simulink model "Final_Dual1"  (R2023a)
settings: Solver=ode113  StartTime=0.0  StopTime=3600  FixedStep=0.01  MaxStep=0.1  RelTol=1e-3
libraries: simulink x3784, slpidlib x2
(part 15 of 158)

== system Final_Dual1/Battery1/Module2/SubModule_4/Cell9 ==
  Cell_Current : Inport
  2RC : Subsystem
  Add : Sum  Inputs=---+
  Lookup Table Dynamic2 : simulink/Lookup Tables/Lookup Table Dynamic  LookUpMeth=Interpolation-Use End Values  OutDataType=fixdt('double')  OutScaling=[]  OutputDataTypeScalingMode=Specify via dialog  OutDataTypeStr=fixdt('double')  DoSatur=off
  Product : Product
  Redution_factor : Constant  Value=[0.8 0.85 0.88 0.95 1 0.98 0.95]
  SOCEstimator : Subsystem  TreatAsAtomicUnit=on
  SOC_Mapping : Subsystem
  Scope : Scope
  Scope1 : Scope
  Scope2 : Scope
  Subsystem : Subsystem
  Temp : Constant  Value=[0 10 20 30 40 50 60]
  Cell_Voltage : Outport
  Cell_temp : Outport  Port=2
  wires:
  2RC/2(V2) -> Add/2
  SOC_Mapping/3(C1) -> 2RC/4(C1)
  SOCEstimator/1(SOC) -> SOC_Mapping/1(SOC), Scope/1
  Add/1 -> Scope2/1, Cell_Voltage/1
  SOC_Mapping/1(Ri) -> Subsystem/2(Ri), 2RC/2(Ri)
  2RC/1(V1) -> Add/1
  2RC/3(Vi) -> Add/3
  Cell_Current/1 -> Subsystem/1(Cell_Current), 2RC/1(Current), SOCEstimator/2(Current)
  SOC_Mapping/2(R1) -> 2RC/3(R1)
  [Cell_Capacity] -> Product/1
  SOC_Mapping/5(C2) -> 2RC/6(C2)
  SOC_Mapping/4(R2) -> 2RC/5(R2)
  [SOC_Iinitial] -> SOCEstimator/1(SOC_Initial)
  SOC_Mapping/6(OCV) -> Add/4
  Subsystem/1(Temp_Cell) -> Scope1/1, SOC_Mapping/2(Cell_Temp), Lookup Table Dynamic2/1, Cell_temp/1
  Product/1 -> SOCEstimator/3(Cell_Capacity)
  Lookup Table Dynamic2/1 -> Product/2
  Temp/1 -> Lookup Table Dynamic2/2
  Redution_factor/1 -> Lookup Table Dynamic2/3

== system Final_Dual1/Battery1/Module2/SubModule_5/Cell1 ==
  Cell_Current : Inport
  2RC : Subsystem
  Add : Sum  Inputs=---+
  Lookup Table Dynamic2 : simulink/Lookup Tables/Lookup Table Dynamic  LookUpMeth=Interpolation-Use End Values  OutDataType=fixdt('double')  OutScaling=[]  OutputDataTypeScalingMode=Specify via dialog  OutDataTypeStr=fixdt('double')  DoSatur=off
  Product : Product
  Redution_factor : Constant  Value=[0.8 0.85 0.88 0.95 1 0.98 0.95]
  SOCEstimator : Subsystem  TreatAsAtomicUnit=on
  SOC_Mapping : Subsystem
  Scope : Scope
  Scope1 : Scope
  Scope2 : Scope
  Subsystem : Subsystem
  Temp : Constant  Value=[0 10 20 30 40 50 60]
  Cell_Voltage : Outport
  Cell_temp : Outport  Port=2
  wires:
  2RC/2(V2) -> Add/2
  SOC_Mapping/3(C1) -> 2RC/4(C1)
  SOCEstimator/1(SOC) -> SOC_Mapping/1(SOC), Scope/1
  Add/1 -> Scope2/1, Cell_Voltage/1
  SOC_Mapping/1(Ri) -> Subsystem/2(Ri), 2RC/2(Ri)
  2RC/1(V1) -> Add/1
  2RC/3(Vi) -> Add/3
  Cell_Current/1 -> Subsystem/1(Cell_Current), 2RC/1(Current), SOCEstimator/2(Current)
  SOC_Mapping/2(R1) -> 2RC/3(R1)
  [Cell_Capacity] -> Product/1
  SOC_Mapping/5(C2) -> 2RC/6(C2)
  SOC_Mapping/4(R2) -> 2RC/5(R2)
  [SOC_Iinitial] -> SOCEstimator/1(SOC_Initial)
  SOC_Mapping/6(OCV) -> Add/4
  Subsystem/1(Temp_Cell) -> Scope1/1, SOC_Mapping/2(Cell_Temp), Lookup Table Dynamic2/1, Cell_temp/1
  Product/1 -> SOCEstimator/3(Cell_Capacity)
  Lookup Table Dynamic2/1 -> Product/2
  Temp/1 -> Lookup Table Dynamic2/2
  Redution_factor/1 -> Lookup Table Dynamic2/3

== system Final_Dual1/Battery1/Module2/SubModule_5/Cell10 ==
  Cell_Current : Inport
  2RC : Subsystem
  Add : Sum  Inputs=---+
  Lookup Table Dynamic2 : simulink/Lookup Tables/Lookup Table Dynamic  LookUpMeth=Interpolation-Use End Values  OutDataType=fixdt('double')  OutScaling=[]  OutputDataTypeScalingMode=Specify via dialog  OutDataTypeStr=fixdt('double')  DoSatur=off
  Product : Product
  Redution_factor : Constant  Value=[0.8 0.85 0.88 0.95 1 0.98 0.95]
  SOCEstimator : Subsystem  TreatAsAtomicUnit=on
  SOC_Mapping : Subsystem
  Scope : Scope
  Scope1 : Scope
  Scope2 : Scope
  Subsystem : Subsystem
  Temp : Constant  Value=[0 10 20 30 40 50 60]
  Cell_Voltage : Outport
  Cell_temp : Outport  Port=2
  wires:
  2RC/2(V2) -> Add/2
  SOC_Mapping/3(C1) -> 2RC/4(C1)
  SOCEstimator/1(SOC) -> SOC_Mapping/1(SOC), Scope/1
  Add/1 -> Scope2/1, Cell_Voltage/1
  SOC_Mapping/1(Ri) -> Subsystem/2(Ri), 2RC/2(Ri)
  2RC/1(V1) -> Add/1
  2RC/3(Vi) -> Add/3
  Cell_Current/1 -> Subsystem/1(Cell_Current), 2RC/1(Current), SOCEstimator/2(Current)
  SOC_Mapping/2(R1) -> 2RC/3(R1)
  [Cell_Capacity] -> Product/1
  SOC_Mapping/5(C2) -> 2RC/6(C2)
  SOC_Mapping/4(R2) -> 2RC/5(R2)
  [SOC_Iinitial] -> SOCEstimator/1(SOC_Initial)
  SOC_Mapping/6(OCV) -> Add/4
  Subsystem/1(Temp_Cell) -> Scope1/1, SOC_Mapping/2(Cell_Temp), Lookup Table Dynamic2/1, Cell_temp/1
  Product/1 -> SOCEstimator/3(Cell_Capacity)
  Lookup Table Dynamic2/1 -> Product/2
  Temp/1 -> Lookup Table Dynamic2/2
  Redution_factor/1 -> Lookup Table Dynamic2/3

== system Final_Dual1/Battery1/Module2/SubModule_5/Cell11 ==
  Cell_Current : Inport
  2RC : Subsystem
  Add : Sum  Inputs=---+
  Lookup Table Dynamic2 : simulink/Lookup Tables/Lookup Table Dynamic  LookUpMeth=Interpolation-Use End Values  OutDataType=fixdt('double')  OutScaling=[]  OutputDataTypeScalingMode=Specify via dialog  OutDataTypeStr=fixdt('double')  DoSatur=off
  Product : Product
  Redution_factor : Constant  Value=[0.8 0.85 0.88 0.95 1 0.98 0.95]
  SOCEstimator : Subsystem  TreatAsAtomicUnit=on
  SOC_Mapping : Subsystem
  Scope : Scope
  Scope1 : Scope
  Scope2 : Scope
  Subsystem : Subsystem
  Temp : Constant  Value=[0 10 20 30 40 50 60]
  Cell_Voltage : Outport
  Cell_temp : Outport  Port=2
  wires:
  Redution_factor/1 -> Lookup Table Dynamic2/3
  Temp/1 -> Lookup Table Dynamic2/2
  Lookup Table Dynamic2/1 -> Product/2
  Product/1 -> SOCEstimator/3(Cell_Capacity)
  Subsystem/1(Temp_Cell) -> Cell_temp/1, Lookup Table Dynamic2/1, SOC_Mapping/2(Cell_Temp), Scope1/1
  SOC_Mapping/6(OCV) -> Add/4
  [SOC_Iinitial] -> SOCEstimator/1(SOC_Initial)
  SOC_Mapping/4(R2) -> 2RC/5(R2)
  SOC_Mapping/5(C2) -> 2RC/6(C2)
  [Cell_Capacity] -> Product/1
  SOC_Mapping/2(R1) -> 2RC/3(R1)
  Cell_Current/1 -> SOCEstimator/2(Current), 2RC/1(Current), Subsystem/1(Cell_Current)
  2RC/3(Vi) -> Add/3
  2RC/1(V1) -> Add/1
  SOC_Mapping/1(Ri) -> 2RC/2(Ri), Subsystem/2(Ri)
  Add/1 -> Cell_Voltage/1, Scope2/1
  SOCEstimator/1(SOC) -> Scope/1, SOC_Mapping/1(SOC)
  SOC_Mapping/3(C1) -> 2RC/4(C1)
  2RC/2(V2) -> Add/2

== system Final_Dual1/Battery1/Module2/SubModule_5/Cell12 ==
  Cell_Current : Inport
  2RC : Subsystem
  Add : Sum  Inputs=---+
  Lookup Table Dynamic2 : simulink/Lookup Tables/Lookup Table Dynamic  LookUpMeth=Interpolation-Use End Values  OutDataType=fixdt('double')  OutScaling=[]  OutputDataTypeScalingMode=Specify via dialog  OutDataTypeStr=fixdt('double')  DoSatur=off
  Product : Product
  Redution_factor : Constant  Value=[0.8 0.85 0.88 0.95 1 0.98 0.95]
  SOCEstimator : Subsystem  TreatAsAtomicUnit=on
  SOC_Mapping : Subsystem
  Scope : Scope
  Scope1 : Scope
  Scope2 : Scope
  Subsystem : Subsystem
  Temp : Constant  Value=[0 10 20 30 40 50 60]
  Cell_Voltage : Outport
  Cell_temp : Outport  Port=2
  wires:
  2RC/2(V2) -> Add/2
  SOC_Mapping/3(C1) -> 2RC/4(C1)
  SOCEstimator/1(SOC) -> SOC_Mapping/1(SOC), Scope/1
  Add/1 -> Scope2/1, Cell_Voltage/1
  SOC_Mapping/1(Ri) -> Subsystem/2(Ri), 2RC/2(Ri)
  2RC/1(V1) -> Add/1
  2RC/3(Vi) -> Add/3
  Cell_Current/1 -> Subsystem/1(Cell_Current), 2RC/1(Current), SOCEstimator/2(Current)
  SOC_Mapping/2(R1) -> 2RC/3(R1)
  [Cell_Capacity] -> Product/1
  SOC_Mapping/5(C2) -> 2RC/6(C2)
  SOC_Mapping/4(R2) -> 2RC/5(R2)
  [SOC_Iinitial] -> SOCEstimator/1(SOC_Initial)
  SOC_Mapping/6(OCV) -> Add/4
  Subsystem/1(Temp_Cell) -> Scope1/1, SOC_Mapping/2(Cell_Temp), Lookup Table Dynamic2/1, Cell_temp/1
  Product/1 -> SOCEstimator/3(Cell_Capacity)
  Lookup Table Dynamic2/1 -> Product/2
  Temp/1 -> Lookup Table Dynamic2/2
  Redution_factor/1 -> Lookup Table Dynamic2/3

== system Final_Dual1/Battery1/Module2/SubModule_5/Cell13 ==
  Cell_Current : Inport
  2RC : Subsystem
  Add : Sum  Inputs=---+
  Lookup Table Dynamic2 : simulink/Lookup Tables/Lookup Table Dynamic  LookUpMeth=Interpolation-Use End Values  OutDataType=fixdt('double')  OutScaling=[]  OutputDataTypeScalingMode=Specify via dialog  OutDataTypeStr=fixdt('double')  DoSatur=off
  Product : Product
  Redution_factor : Constant  Value=[0.8 0.85 0.88 0.95 1 0.98 0.95]
  SOCEstimator : Subsystem  TreatAsAtomicUnit=on
  SOC_Mapping : Subsystem
  Scope : Scope
  Scope1 : Scope
  Scope2 : Scope
  Subsystem : Subsystem
  Temp : Constant  Value=[0 10 20 30 40 50 60]
  Cell_Voltage : Outport
  Cell_temp : Outport  Port=2
  wires:
  Redution_factor/1 -> Lookup Table Dynamic2/3
  Temp/1 -> Lookup Table Dynamic2/2
  Lookup Table Dynamic2/1 -> Product/2
  Product/1 -> SOCEstimator/3(Cell_Capacity)
  Subsystem/1(Temp_Cell) -> Cell_temp/1, Lookup Table Dynamic2/1, SOC_Mapping/2(Cell_Temp), Scope1/1
  SOC_Mapping/6(OCV) -> Add/4
  [SOC_Iinitial] -> SOCEstimator/1(SOC_Initial)
  SOC_Mapping/4(R2) -> 2RC/5(R2)
  SOC_Mapping/5(C2) -> 2RC/6(C2)
  [Cell_Capacity] -> Product/1
  SOC_Mapping/2(R1) -> 2RC/3(R1)
  Cell_Current/1 -> SOCEstimator/2(Current), 2RC/1(Current), Subsystem/1(Cell_Current)
  2RC/3(Vi) -> Add/3
  2RC/1(V1) -> Add/1
  SOC_Mapping/1(Ri) -> 2RC/2(Ri), Subsystem/2(Ri)
  Add/1 -> Cell_Voltage/1, Scope2/1
  SOCEstimator/1(SOC) -> Scope/1, SOC_Mapping/1(SOC)
  SOC_Mapping/3(C1) -> 2RC/4(C1)
  2RC/2(V2) -> Add/2

== system Final_Dual1/Battery1/Module2/SubModule_5/Cell14 ==
  Cell_Current : Inport
  2RC : Subsystem
  Add : Sum  Inputs=---+
  Lookup Table Dynamic2 : simulink/Lookup Tables/Lookup Table Dynamic  LookUpMeth=Interpolation-Use End Values  OutDataType=fixdt('double')  OutScaling=[]  OutputDataTypeScalingMode=Specify via dialog  OutDataTypeStr=fixdt('double')  DoSatur=off
  Product : Product
  Redution_factor : Constant  Value=[0.8 0.85 0.88 0.95 1 0.98 0.95]
  SOCEstimator : Subsystem  TreatAsAtomicUnit=on
  SOC_Mapping : Subsystem
  Scope : Scope
  Scope1 : Scope
  Scope2 : Scope
  Subsystem : Subsystem
  Temp : Constant  Value=[0 10 20 30 40 50 60]
  Cell_Voltage : Outport
  Cell_temp : Outport  Port=2
  wires:
  Redution_factor/1 -> Lookup Table Dynamic2/3
  Temp/1 -> Lookup Table Dynamic2/2
  Lookup Table Dynamic2/1 -> Product/2
  Product/1 -> SOCEstimator/3(Cell_Capacity)
  Subsystem/1(Temp_Cell) -> Cell_temp/1, Lookup Table Dynamic2/1, SOC_Mapping/2(Cell_Temp), Scope1/1
  SOC_Mapping/6(OCV) -> Add/4
  [SOC_Iinitial] -> SOCEstimator/1(SOC_Initial)
  SOC_Mapping/4(R2) -> 2RC/5(R2)
  SOC_Mapping/5(C2) -> 2RC/6(C2)
  [Cell_Capacity] -> Product/1
  SOC_Mapping/2(R1) -> 2RC/3(R1)
  Cell_Current/1 -> SOCEstimator/2(Current), 2RC/1(Current), Subsystem/1(Cell_Current)
  2RC/3(Vi) -> Add/3
  2RC/1(V1) -> Add/1
  SOC_Mapping/1(Ri) -> 2RC/2(Ri), Subsystem/2(Ri)
  Add/1 -> Cell_Voltage/1, Scope2/1
  SOCEstimator/1(SOC) -> Scope/1, SOC_Mapping/1(SOC)
  SOC_Mapping/3(C1) -> 2RC/4(C1)
  2RC/2(V2) -> Add/2

== system Final_Dual1/Battery1/Module2/SubModule_5/Cell15 ==
  Cell_Current : Inport
  2RC : Subsystem
  Add : Sum  Inputs=---+
  Lookup Table Dynamic2 : simulink/Lookup Tables/Lookup Table Dynamic  LookUpMeth=Interpolation-Use End Values  OutDataType=fixdt('double')  OutScaling=[]  OutputDataTypeScalingMode=Specify via dialog  OutDataTypeStr=fixdt('double')  DoSatur=off
  Product : Product
  Redution_factor : Constant  Value=[0.8 0.85 0.88 0.95 1 0.98 0.95]
  SOCEstimator : Subsystem  TreatAsAtomicUnit=on
  SOC_Mapping : Subsystem
  Scope : Scope
  Scope1 : Scope
  Scope2 : Scope
  Subsystem : Subsystem
  Temp : Constant  Value=[0 10 20 30 40 50 60]
  Cell_Voltage : Outport
  Cell_temp : Outport  Port=2
  wires:
  Redution_factor/1 -> Lookup Table Dynamic2/3
  Temp/1 -> Lookup Table Dynamic2/2
  Lookup Table Dynamic2/1 -> Product/2
  Product/1 -> SOCEstimator/3(Cell_Capacity)
  Subsystem/1(Temp_Cell) -> Cell_temp/1, Lookup Table Dynamic2/1, SOC_Mapping/2(Cell_Temp), Scope1/1
  SOC_Mapping/6(OCV) -> Add/4
  [SOC_Iinitial] -> SOCEstimator/1(SOC_Initial)
  SOC_Mapping/4(R2) -> 2RC/5(R2)
  SOC_Mapping/5(C2) -> 2RC/6(C2)
  [Cell_Capacity] -> Product/1
  SOC_Mapping/2(R1) -> 2RC/3(R1)
  Cell_Current/1 -> SOCEstimator/2(Current), 2RC/1(Current), Subsystem/1(Cell_Current)
  2RC/3(Vi) -> Add/3
  2RC/1(V1) -> Add/1
  SOC_Mapping/1(Ri) -> 2RC/2(Ri), Subsystem/2(Ri)
  Add/1 -> Cell_Voltage/1, Scope2/1
  SOCEstimator/1(SOC) -> Scope/1, SOC_Mapping/1(SOC)
  SOC_Mapping/3(C1) -> 2RC/4(C1)
  2RC/2(V2) -> Add/2

== system Final_Dual1/Battery1/Module2/SubModule_5/Cell16 ==
  Cell_Current : Inport
  2RC : Subsystem
  Add : Sum  Inputs=---+
  Lookup Table Dynamic2 : simulink/Lookup Tables/Lookup Table Dynamic  LookUpMeth=Interpolation-Use End Values  OutDataType=fixdt('double')  OutScaling=[]  OutputDataTypeScalingMode=Specify via dialog  OutDataTypeStr=fixdt('double')  DoSatur=off
  Product : Product
  Redution_factor : Constant  Value=[0.8 0.85 0.88 0.95 1 0.98 0.95]
  SOCEstimator : Subsystem  TreatAsAtomicUnit=on
  SOC_Mapping : Subsystem
  Scope : Scope
  Scope1 : Scope
  Scope2 : Scope
  Subsystem : Subsystem
  Temp : Constant  Value=[0 10 20 30 40 50 60]
  Cell_Voltage : Outport
  Cell_temp : Outport  Port=2
  wires:
  Redution_factor/1 -> Lookup Table Dynamic2/3
  Temp/1 -> Lookup Table Dynamic2/2
  Lookup Table Dynamic2/1 -> Product/2
  Product/1 -> SOCEstimator/3(Cell_Capacity)
  Subsystem/1(Temp_Cell) -> Cell_temp/1, Lookup Table Dynamic2/1, SOC_Mapping/2(Cell_Temp), Scope1/1
  SOC_Mapping/6(OCV) -> Add/4
  [SOC_Iinitial] -> SOCEstimator/1(SOC_Initial)
  SOC_Mapping/4(R2) -> 2RC/5(R2)
  SOC_Mapping/5(C2) -> 2RC/6(C2)
  [Cell_Capacity] -> Product/1
  SOC_Mapping/2(R1) -> 2RC/3(R1)
  Cell_Current/1 -> SOCEstimator/2(Current), 2RC/1(Current), Subsystem/1(Cell_Current)
  2RC/3(Vi) -> Add/3
  2RC/1(V1) -> Add/1
  SOC_Mapping/1(Ri) -> 2RC/2(Ri), Subsystem/2(Ri)
  Add/1 -> Cell_Voltage/1, Scope2/1
  SOCEstimator/1(SOC) -> Scope/1, SOC_Mapping/1(SOC)
  SOC_Mapping/3(C1) -> 2RC/4(C1)
  2RC/2(V2) -> Add/2

== system Final_Dual1/Battery1/Module2/SubModule_5/Cell17 ==
  Cell_Current : Inport
  2RC : Subsystem
  Add : Sum  Inputs=---+
  Lookup Table Dynamic2 : simulink/Lookup Tables/Lookup Table Dynamic  LookUpMeth=Interpolation-Use End Values  OutDataType=fixdt('double')  OutScaling=[]  OutputDataTypeScalingMode=Specify via dialog  OutDataTypeStr=fixdt('double')  DoSatur=off
  Product : Product
  Redution_factor : Constant  Value=[0.8 0.85 0.88 0.95 1 0.98 0.95]
  SOCEstimator : Subsystem  TreatAsAtomicUnit=on
  SOC_Mapping : Subsystem
  Scope : Scope
  Scope1 : Scope
  Scope2 : Scope
  Subsystem : Subsystem
  Temp : Constant  Value=[0 10 20 30 40 50 60]
  Cell_Voltage : Outport
  Cell_temp : Outport  Port=2
  wires:
  2RC/2(V2) -> Add/2
  SOC_Mapping/3(C1) -> 2RC/4(C1)
  SOCEstimator/1(SOC) -> SOC_Mapping/1(SOC), Scope/1
  Add/1 -> Scope2/1, Cell_Voltage/1
  SOC_Mapping/1(Ri) -> Subsystem/2(Ri), 2RC/2(Ri)
  2RC/1(V1) -> Add/1
  2RC/3(Vi) -> Add/3
  Cell_Current/1 -> Subsystem/1(Cell_Current), 2RC/1(Current), SOCEstimator/2(Current)
  SOC_Mapping/2(R1) -> 2RC/3(R1)
  [Cell_Capacity] -> Product/1
  SOC_Mapping/5(C2) -> 2RC/6(C2)
  SOC_Mapping/4(R2) -> 2RC/5(R2)
  [SOC_Iinitial] -> SOCEstimator/1(SOC_Initial)
  SOC_Mapping/6(OCV) -> Add/4
  Subsystem/1(Temp_Cell) -> Scope1/1, SOC_Mapping/2(Cell_Temp), Lookup Table Dynamic2/1, Cell_temp/1
  Product/1 -> SOCEstimator/3(Cell_Capacity)
  Lookup Table Dynamic2/1 -> Product/2
  Temp/1 -> Lookup Table Dynamic2/2
  Redution_factor/1 -> Lookup Table Dynamic2/3

== system Final_Dual1/Battery1/Module2/SubModule_5/Cell18 ==
  Cell_Current : Inport
  2RC : Subsystem
  Add : Sum  Inputs=---+
  Lookup Table Dynamic2 : simulink/Lookup Tables/Lookup Table Dynamic  LookUpMeth=Interpolation-Use End Values  OutDataType=fixdt('double')  OutScaling=[]  OutputDataTypeScalingMode=Specify via dialog  OutDataTypeStr=fixdt('double')  DoSatur=off
  Product : Product
  Redution_factor : Constant  Value=[0.8 0.85 0.88 0.95 1 0.98 0.95]
  SOCEstimator : Subsystem  TreatAsAtomicUnit=on
  SOC_Mapping : Subsystem
  Scope : Scope
  Scope1 : Scope
  Scope2 : Scope
  Subsystem : Subsystem
  Temp : Constant  Value=[0 10 20 30 40 50 60]
  Cell_Voltage : Outport
  Cell_temp : Outport  Port=2
  wires:
  Redution_factor/1 -> Lookup Table Dynamic2/3
  Temp/1 -> Lookup Table Dynamic2/2
  Lookup Table Dynamic2/1 -> Product/2
  Product/1 -> SOCEstimator/3(Cell_Capacity)
  Subsystem/1(Temp_Cell) -> Cell_temp/1, Lookup Table Dynamic2/1, SOC_Mapping/2(Cell_Temp), Scope1/1
  SOC_Mapping/6(OCV) -> Add/4
  [SOC_Iinitial] -> SOCEstimator/1(SOC_Initial)
  SOC_Mapping/4(R2) -> 2RC/5(R2)
  SOC_Mapping/5(C2) -> 2RC/6(C2)
  [Cell_Capacity] -> Product/1
  SOC_Mapping/2(R1) -> 2RC/3(R1)
  Cell_Current/1 -> SOCEstimator/2(Current), 2RC/1(Current), Subsystem/1(Cell_Current)
  2RC/3(Vi) -> Add/3
  2RC/1(V1) -> Add/1
  SOC_Mapping/1(Ri) -> 2RC/2(Ri), Subsystem/2(Ri)
  Add/1 -> Cell_Voltage/1, Scope2/1
  SOCEstimator/1(SOC) -> Scope/1, SOC_Mapping/1(SOC)
  SOC_Mapping/3(C1) -> 2RC/4(C1)
  2RC/2(V2) -> Add/2

== system Final_Dual1/Battery1/Module2/SubModule_5/Cell19 ==
  Cell_Current : Inport
  2RC : Subsystem
  Add : Sum  Inputs=---+
  Lookup Table Dynamic2 : simulink/Lookup Tables/Lookup Table Dynamic  LookUpMeth=Interpolation-Use End Values  OutDataType=fixdt('double')  OutScaling=[]  OutputDataTypeScalingMode=Specify via dialog  OutDataTypeStr=fixdt('double')  DoSatur=off
  Product : Product
  Redution_factor : Constant  Value=[0.8 0.85 0.88 0.95 1 0.98 0.95]
  SOCEstimator : Subsystem  TreatAsAtomicUnit=on
  SOC_Mapping : Subsystem
  Scope : Scope
  Scope1 : Scope
  Scope2 : Scope
  Subsystem : Subsystem
  Temp : Constant  Value=[0 10 20 30 40 50 60]
  Cell_Voltage : Outport
  Cell_temp : Outport  Port=2
  wires:
  2RC/2(V2) -> Add/2
  SOC_Mapping/3(C1) -> 2RC/4(C1)
  SOCEstimator/1(SOC) -> SOC_Mapping/1(SOC), Scope/1
  Add/1 -> Scope2/1, Cell_Voltage/1
  SOC_Mapping/1(Ri) -> Subsystem/2(Ri), 2RC/2(Ri)
  2RC/1(V1) -> Add/1
  2RC/3(Vi) -> Add/3
  Cell_Current/1 -> Subsystem/1(Cell_Current), 2RC/1(Current), SOCEstimator/2(Current)
  SOC_Mapping/2(R1) -> 2RC/3(R1)
  [Cell_Capacity] -> Product/1
  SOC_Mapping/5(C2) -> 2RC/6(C2)
  SOC_Mapping/4(R2) -> 2RC/5(R2)
  [SOC_Iinitial] -> SOCEstimator/1(SOC_Initial)
  SOC_Mapping/6(OCV) -> Add/4
  Subsystem/1(Temp_Cell) -> Scope1/1, SOC_Mapping/2(Cell_Temp), Lookup Table Dynamic2/1, Cell_temp/1
  Product/1 -> SOCEstimator/3(Cell_Capacity)
  Lookup Table Dynamic2/1 -> Product/2
  Temp/1 -> Lookup Table Dynamic2/2
  Redution_factor/1 -> Lookup Table Dynamic2/3

== system Final_Dual1/Battery1/Module2/SubModule_5/Cell2 ==
  Cell_Current : Inport
  2RC : Subsystem
  Add : Sum  Inputs=---+
  Lookup Table Dynamic2 : simulink/Lookup Tables/Lookup Table Dynamic  LookUpMeth=Interpolation-Use End Values  OutDataType=fixdt('double')  OutScaling=[]  OutputDataTypeScalingMode=Specify via dialog  OutDataTypeStr=fixdt('double')  DoSatur=off
  Product : Product
  Redution_factor : Constant  Value=[0.8 0.85 0.88 0.95 1 0.98 0.95]
  SOCEstimator : Subsystem  TreatAsAtomicUnit=on
  SOC_Mapping : Subsystem
  Scope : Scope
  Scope1 : Scope
  Scope2 : Scope
  Subsystem : Subsystem
  Temp : Constant  Value=[0 10 20 30 40 50 60]
  Cell_Voltage : Outport
  Cell_temp : Outport  Port=2
  wires:
  Redution_factor/1 -> Lookup Table Dynamic2/3
  Temp/1 -> Lookup Table Dynamic2/2
  Lookup Table Dynamic2/1 -> Product/2
  Product/1 -> SOCEstimator/3(Cell_Capacity)
  Subsystem/1(Temp_Cell) -> Cell_temp/1, Lookup Table Dynamic2/1, SOC_Mapping/2(Cell_Temp), Scope1/1
  SOC_Mapping/6(OCV) -> Add/4
  [SOC_Iinitial] -> SOCEstimator/1(SOC_Initial)
  SOC_Mapping/4(R2) -> 2RC/5(R2)
  SOC_Mapping/5(C2) -> 2RC/6(C2)
  [Cell_Capacity] -> Product/1
  SOC_Mapping/2(R1) -> 2RC/3(R1)
  Cell_Current/1 -> SOCEstimator/2(Current), 2RC/1(Current), Subsystem/1(Cell_Current)
  2RC/3(Vi) -> Add/3
  2RC/1(V1) -> Add/1
  SOC_Mapping/1(Ri) -> 2RC/2(Ri), Subsystem/2(Ri)
  Add/1 -> Cell_Voltage/1, Scope2/1
  SOCEstimator/1(SOC) -> Scope/1, SOC_Mapping/1(SOC)
  SOC_Mapping/3(C1) -> 2RC/4(C1)
  2RC/2(V2) -> Add/2

== system Final_Dual1/Battery1/Module2/SubModule_5/Cell20 ==
  Cell_Current : Inport
  2RC : Subsystem
  Add : Sum  Inputs=---+
  Lookup Table Dynamic2 : simulink/Lookup Tables/Lookup Table Dynamic  LookUpMeth=Interpolation-Use End Values  OutDataType=fixdt('double')  OutScaling=[]  OutputDataTypeScalingMode=Specify via dialog  OutDataTypeStr=fixdt('double')  DoSatur=off
  Product : Product
  Redution_factor : Constant  Value=[0.8 0.85 0.88 0.95 1 0.98 0.95]
  SOCEstimator : Subsystem  TreatAsAtomicUnit=on
  SOC_Mapping : Subsystem
  Scope : Scope
  Scope1 : Scope
  Scope2 : Scope
  Subsystem : Subsystem
  Temp : Constant  Value=[0 10 20 30 40 50 60]
  Cell_Voltage : Outport
  Cell_temp : Outport  Port=2
  wires:
  Redution_factor/1 -> Lookup Table Dynamic2/3
  Temp/1 -> Lookup Table Dynamic2/2
  Lookup Table Dynamic2/1 -> Product/2
  Product/1 -> SOCEstimator/3(Cell_Capacity)
  Subsystem/1(Temp_Cell) -> Cell_temp/1, Lookup Table Dynamic2/1, SOC_Mapping/2(Cell_Temp), Scope1/1
  SOC_Mapping/6(OCV) -> Add/4
  [SOC_Iinitial] -> SOCEstimator/1(SOC_Initial)
  SOC_Mapping/4(R2) -> 2RC/5(R2)
  SOC_Mapping/5(C2) -> 2RC/6(C2)
  [Cell_Capacity] -> Product/1
  SOC_Mapping/2(R1) -> 2RC/3(R1)
  Cell_Current/1 -> SOCEstimator/2(Current), 2RC/1(Current), Subsystem/1(Cell_Current)
  2RC/3(Vi) -> Add/3
  2RC/1(V1) -> Add/1
  SOC_Mapping/1(Ri) -> 2RC/2(Ri), Subsystem/2(Ri)
  Add/1 -> Cell_Voltage/1, Scope2/1
  SOCEstimator/1(SOC) -> Scope/1, SOC_Mapping/1(SOC)
  SOC_Mapping/3(C1) -> 2RC/4(C1)
  2RC/2(V2) -> Add/2

== system Final_Dual1/Battery1/Module2/SubModule_5/Cell21 ==
  Cell_Current : Inport
  2RC : Subsystem
  Add : Sum  Inputs=---+
  Lookup Table Dynamic2 : simulink/Lookup Tables/Lookup Table Dynamic  LookUpMeth=Interpolation-Use End Values  OutDataType=fixdt('double')  OutScaling=[]  OutputDataTypeScalingMode=Specify via dialog  OutDataTypeStr=fixdt('double')  DoSatur=off
  Product : Product
  Redution_factor : Constant  Value=[0.8 0.85 0.88 0.95 1 0.98 0.95]
  SOCEstimator : Subsystem  TreatAsAtomicUnit=on
  SOC_Mapping : Subsystem
  Scope : Scope
  Scope1 : Scope
  Scope2 : Scope
  Subsystem : Subsystem
  Temp : Constant  Value=[0 10 20 30 40 50 60]
  Cell_Voltage : Outport
  Cell_temp : Outport  Port=2
  wires:
  2RC/2(V2) -> Add/2
  SOC_Mapping/3(C1) -> 2RC/4(C1)
  SOCEstimator/1(SOC) -> SOC_Mapping/1(SOC), Scope/1
  Add/1 -> Scope2/1, Cell_Voltage/1
  SOC_Mapping/1(Ri) -> Subsystem/2(Ri), 2RC/2(Ri)
  2RC/1(V1) -> Add/1
  2RC/3(Vi) -> Add/3
  Cell_Current/1 -> Subsystem/1(Cell_Current), 2RC/1(Current), SOCEstimator/2(Current)
  SOC_Mapping/2(R1) -> 2RC/3(R1)
  [Cell_Capacity] -> Product/1
  SOC_Mapping/5(C2) -> 2RC/6(C2)
  SOC_Mapping/4(R2) -> 2RC/5(R2)
  [SOC_Iinitial] -> SOCEstimator/1(SOC_Initial)
  SOC_Mapping/6(OCV) -> Add/4
  Subsystem/1(Temp_Cell) -> Scope1/1, SOC_Mapping/2(Cell_Temp), Lookup Table Dynamic2/1, Cell_temp/1
  Product/1 -> SOCEstimator/3(Cell_Capacity)
  Lookup Table Dynamic2/1 -> Product/2
  Temp/1 -> Lookup Table Dynamic2/2
  Redution_factor/1 -> Lookup Table Dynamic2/3

== system Final_Dual1/Battery1/Module2/SubModule_5/Cell22 ==
  Cell_Current : Inport
  2RC : Subsystem
  Add : Sum  Inputs=---+
  Lookup Table Dynamic2 : simulink/Lookup Tables/Lookup Table Dynamic  LookUpMeth=Interpolation-Use End Values  OutDataType=fixdt('double')  OutScaling=[]  OutputDataTypeScalingMode=Specify via dialog  OutDataTypeStr=fixdt('double')  DoSatur=off
  Product : Product
  Redution_factor : Constant  Value=[0.8 0.85 0.88 0.95 1 0.98 0.95]
  SOCEstimator : Subsystem  TreatAsAtomicUnit=on
  SOC_Mapping : Subsystem
  Scope : Scope
  Scope1 : Scope
  Scope2 : Scope
  Subsystem : Subsystem
  Temp : Constant  Value=[0 10 20 30 40 50 60]
  Cell_Voltage : Outport
  Cell_temp : Outport  Port=2
  wires:
  2RC/2(V2) -> Add/2
  SOC_Mapping/3(C1) -> 2RC/4(C1)
  SOCEstimator/1(SOC) -> SOC_Mapping/1(SOC), Scope/1
  Add/1 -> Scope2/1, Cell_Voltage/1
  SOC_Mapping/1(Ri) -> Subsystem/2(Ri), 2RC/2(Ri)
  2RC/1(V1) -> Add/1
  2RC/3(Vi) -> Add/3
  Cell_Current/1 -> Subsystem/1(Cell_Current), 2RC/1(Current), SOCEstimator/2(Current)
  SOC_Mapping/2(R1) -> 2RC/3(R1)
  [Cell_Capacity] -> Product/1
  SOC_Mapping/5(C2) -> 2RC/6(C2)
  SOC_Mapping/4(R2) -> 2RC/5(R2)
  [SOC_Iinitial] -> SOCEstimator/1(SOC_Initial)
  SOC_Mapping/6(OCV) -> Add/4
  Subsystem/1(Temp_Cell) -> Scope1/1, SOC_Mapping/2(Cell_Temp), Lookup Table Dynamic2/1, Cell_temp/1
  Product/1 -> SOCEstimator/3(Cell_Capacity)
  Lookup Table Dynamic2/1 -> Product/2
  Temp/1 -> Lookup Table Dynamic2/2
  Redution_factor/1 -> Lookup Table Dynamic2/3

== system Final_Dual1/Battery1/Module2/SubModule_5/Cell3 ==
  Cell_Current : Inport
  2RC : Subsystem
  Add : Sum  Inputs=---+
  Lookup Table Dynamic2 : simulink/Lookup Tables/Lookup Table Dynamic  LookUpMeth=Interpolation-Use End Values  OutDataType=fixdt('double')  OutScaling=[]  OutputDataTypeScalingMode=Specify via dialog  OutDataTypeStr=fixdt('double')  DoSatur=off
  Product : Product
  Redution_factor : Constant  Value=[0.8 0.85 0.88 0.95 1 0.98 0.95]
  SOCEstimator : Subsystem  TreatAsAtomicUnit=on
  SOC_Mapping : Subsystem
  Scope : Scope
  Scope1 : Scope
  Scope2 : Scope
  Subsystem : Subsystem
  Temp : Constant  Value=[0 10 20 30 40 50 60]
  Cell_Voltage : Outport
  Cell_temp : Outport  Port=2
  wires:
  2RC/2(V2) -> Add/2
  SOC_Mapping/3(C1) -> 2RC/4(C1)
  SOCEstimator/1(SOC) -> SOC_Mapping/1(SOC), Scope/1
  Add/1 -> Scope2/1, Cell_Voltage/1
  SOC_Mapping/1(Ri) -> Subsystem/2(Ri), 2RC/2(Ri)
  2RC/1(V1) -> Add/1
  2RC/3(Vi) -> Add/3
  Cell_Current/1 -> Subsystem/1(Cell_Current), 2RC/1(Current), SOCEstimator/2(Current)
  SOC_Mapping/2(R1) -> 2RC/3(R1)
  [Cell_Capacity] -> Product/1
  SOC_Mapping/5(C2) -> 2RC/6(C2)
  SOC_Mapping/4(R2) -> 2RC/5(R2)
  [SOC_Iinitial] -> SOCEstimator/1(SOC_Initial)
  SOC_Mapping/6(OCV) -> Add/4
  Subsystem/1(Temp_Cell) -> Scope1/1, SOC_Mapping/2(Cell_Temp), Lookup Table Dynamic2/1, Cell_temp/1
  Product/1 -> SOCEstimator/3(Cell_Capacity)
  Lookup Table Dynamic2/1 -> Product/2
  Temp/1 -> Lookup Table Dynamic2/2
  Redution_factor/1 -> Lookup Table Dynamic2/3

== system Final_Dual1/Battery1/Module2/SubModule_5/Cell4 ==
  Cell_Current : Inport
  2RC : Subsystem
  Add : Sum  Inputs=---+
  Lookup Table Dynamic2 : simulink/Lookup Tables/Lookup Table Dynamic  LookUpMeth=Interpolation-Use End Values  OutDataType=fixdt('double')  OutScaling=[]  OutputDataTypeScalingMode=Specify via dialog  OutDataTypeStr=fixdt('double')  DoSatur=off
  Product : Product
  Redution_factor : Constant  Value=[0.8 0.85 0.88 0.95 1 0.98 0.95]
  SOCEstimator : Subsystem  TreatAsAtomicUnit=on
  SOC_Mapping : Subsystem
  Scope : Scope
  Scope1 : Scope
  Scope2 : Scope
  Subsystem : Subsystem
  Temp : Constant  Value=[0 10 20 30 40 50 60]
  Cell_Voltage : Outport
  Cell_temp : Outport  Port=2
  wires:
  Redution_factor/1 -> Lookup Table Dynamic2/3
  Temp/1 -> Lookup Table Dynamic2/2
  Lookup Table Dynamic2/1 -> Product/2
  Product/1 -> SOCEstimator/3(Cell_Capacity)
  Subsystem/1(Temp_Cell) -> Cell_temp/1, Lookup Table Dynamic2/1, SOC_Mapping/2(Cell_Temp), Scope1/1
  SOC_Mapping/6(OCV) -> Add/4
  [SOC_Iinitial] -> SOCEstimator/1(SOC_Initial)
  SOC_Mapping/4(R2) -> 2RC/5(R2)
  SOC_Mapping/5(C2) -> 2RC/6(C2)
  [Cell_Capacity] -> Product/1
  SOC_Mapping/2(R1) -> 2RC/3(R1)
  Cell_Current/1 -> SOCEstimator/2(Current), 2RC/1(Current), Subsystem/1(Cell_Current)
  2RC/3(Vi) -> Add/3
  2RC/1(V1) -> Add/1
  SOC_Mapping/1(Ri) -> 2RC/2(Ri), Subsystem/2(Ri)
  Add/1 -> Cell_Voltage/1, Scope2/1
  SOCEstimator/1(SOC) -> Scope/1, SOC_Mapping/1(SOC)
  SOC_Mapping/3(C1) -> 2RC/4(C1)
  2RC/2(V2) -> Add/2

== system Final_Dual1/Battery1/Module2/SubModule_5/Cell5 ==
  Cell_Current : Inport
  2RC : Subsystem
  Add : Sum  Inputs=---+
  Lookup Table Dynamic2 : simulink/Lookup Tables/Lookup Table Dynamic  LookUpMeth=Interpolation-Use End Values  OutDataType=fixdt('double')  OutScaling=[]  OutputDataTypeScalingMode=Specify via dialog  OutDataTypeStr=fixdt('double')  DoSatur=off
  Product : Product
  Redution_factor : Constant  Value=[0.8 0.85 0.88 0.95 1 0.98 0.95]
  SOCEstimator : Subsystem  TreatAsAtomicUnit=on
  SOC_Mapping : Subsystem
  Scope : Scope
  Scope1 : Scope
  Scope2 : Scope
  Subsystem : Subsystem
  Temp : Constant  Value=[0 10 20 30 40 50 60]
  Cell_Voltage : Outport
  Cell_temp : Outport  Port=2
  wires:
  2RC/2(V2) -> Add/2
  SOC_Mapping/3(C1) -> 2RC/4(C1)
  SOCEstimator/1(SOC) -> SOC_Mapping/1(SOC), Scope/1
  Add/1 -> Scope2/1, Cell_Voltage/1
  SOC_Mapping/1(Ri) -> Subsystem/2(Ri), 2RC/2(Ri)
  2RC/1(V1) -> Add/1
  2RC/3(Vi) -> Add/3
  Cell_Current/1 -> Subsystem/1(Cell_Current), 2RC/1(Current), SOCEstimator/2(Current)
  SOC_Mapping/2(R1) -> 2RC/3(R1)
  [Cell_Capacity] -> Product/1
  SOC_Mapping/5(C2) -> 2RC/6(C2)
  SOC_Mapping/4(R2) -> 2RC/5(R2)
  [SOC_Iinitial] -> SOCEstimator/1(SOC_Initial)
  SOC_Mapping/6(OCV) -> Add/4
  Subsystem/1(Temp_Cell) -> Scope1/1, SOC_Mapping/2(Cell_Temp), Lookup Table Dynamic2/1, Cell_temp/1
  Product/1 -> SOCEstimator/3(Cell_Capacity)
  Lookup Table Dynamic2/1 -> Product/2
  Temp/1 -> Lookup Table Dynamic2/2
  Redution_factor/1 -> Lookup Table Dynamic2/3

== system Final_Dual1/Battery1/Module2/SubModule_5/Cell6 ==
  Cell_Current : Inport
  2RC : Subsystem
  Add : Sum  Inputs=---+
  Lookup Table Dynamic2 : simulink/Lookup Tables/Lookup Table Dynamic  LookUpMeth=Interpolation-Use End Values  OutDataType=fixdt('double')  OutScaling=[]  OutputDataTypeScalingMode=Specify via dialog  OutDataTypeStr=fixdt('double')  DoSatur=off
  Product : Product
  Redution_factor : Constant  Value=[0.8 0.85 0.88 0.95 1 0.98 0.95]
  SOCEstimator : Subsystem  TreatAsAtomicUnit=on
  SOC_Mapping : Subsystem
  Scope : Scope
  Scope1 : Scope
  Scope2 : Scope
  Subsystem : Subsystem
  Temp : Constant  Value=[0 10 20 30 40 50 60]
  Cell_Voltage : Outport
  Cell_temp : Outport  Port=2
  wires:
  Redution_factor/1 -> Lookup Table Dynamic2/3
  Temp/1 -> Lookup Table Dynamic2/2
  Lookup Table Dynamic2/1 -> Product/2
  Product/1 -> SOCEstimator/3(Cell_Capacity)
  Subsystem/1(Temp_Cell) -> Cell_temp/1, Lookup Table Dynamic2/1, SOC_Mapping/2(Cell_Temp), Scope1/1
  SOC_Mapping/6(OCV) -> Add/4
  [SOC_Iinitial] -> SOCEstimator/1(SOC_Initial)
  SOC_Mapping/4(R2) -> 2RC/5(R2)
  SOC_Mapping/5(C2) -> 2RC/6(C2)
  [Cell_Capacity] -> Product/1
  SOC_Mapping/2(R1) -> 2RC/3(R1)
  Cell_Current/1 -> SOCEstimator/2(Current), 2RC/1(Current), Subsystem/1(Cell_Current)
  2RC/3(Vi) -> Add/3
  2RC/1(V1) -> Add/1
  SOC_Mapping/1(Ri) -> 2RC/2(Ri), Subsystem/2(Ri)
  Add/1 -> Cell_Voltage/1, Scope2/1
  SOCEstimator/1(SOC) -> Scope/1, SOC_Mapping/1(SOC)
  SOC_Mapping/3(C1) -> 2RC/4(C1)
  2RC/2(V2) -> Add/2

== system Final_Dual1/Battery1/Module2/SubModule_5/Cell7 ==
  Cell_Current : Inport
  2RC : Subsystem
  Add : Sum  Inputs=---+
  Lookup Table Dynamic2 : simulink/Lookup Tables/Lookup Table Dynamic  LookUpMeth=Interpolation-Use End Values  OutDataType=fixdt('double')  OutScaling=[]  OutputDataTypeScalingMode=Specify via dialog  OutDataTypeStr=fixdt('double')  DoSatur=off
  Product : Product
  Redution_factor : Constant  Value=[0.8 0.85 0.88 0.95 1 0.98 0.95]
  SOCEstimator : Subsystem  TreatAsAtomicUnit=on
  SOC_Mapping : Subsystem
  Scope : Scope
  Scope1 : Scope
  Scope2 : Scope
  Subsystem : Subsystem
  Temp : Constant  Value=[0 10 20 30 40 50 60]
  Cell_Voltage : Outport
  Cell_temp : Outport  Port=2
  wires:
  Redution_factor/1 -> Lookup Table Dynamic2/3
  Temp/1 -> Lookup Table Dynamic2/2
  Lookup Table Dynamic2/1 -> Product/2
  Product/1 -> SOCEstimator/3(Cell_Capacity)
  Subsystem/1(Temp_Cell) -> Cell_temp/1, Lookup Table Dynamic2/1, SOC_Mapping/2(Cell_Temp), Scope1/1
  SOC_Mapping/6(OCV) -> Add/4
  [SOC_Iinitial] -> SOCEstimator/1(SOC_Initial)
  SOC_Mapping/4(R2) -> 2RC/5(R2)
  SOC_Mapping/5(C2) -> 2RC/6(C2)
  [Cell_Capacity] -> Product/1
  SOC_Mapping/2(R1) -> 2RC/3(R1)
  Cell_Current/1 -> SOCEstimator/2(Current), 2RC/1(Current), Subsystem/1(Cell_Current)
  2RC/3(Vi) -> Add/3
  2RC/1(V1) -> Add/1
  SOC_Mapping/1(Ri) -> 2RC/2(Ri), Subsystem/2(Ri)
  Add/1 -> Cell_Voltage/1, Scope2/1
  SOCEstimator/1(SOC) -> Scope/1, SOC_Mapping/1(SOC)
  SOC_Mapping/3(C1) -> 2RC/4(C1)
  2RC/2(V2) -> Add/2

== system Final_Dual1/Battery1/Module2/SubModule_5/Cell8 ==
  Cell_Current : Inport
  2RC : Subsystem
  Add : Sum  Inputs=---+
  Lookup Table Dynamic2 : simulink/Lookup Tables/Lookup Table Dynamic  LookUpMeth=Interpolation-Use End Values  OutDataType=fixdt('double')  OutScaling=[]  OutputDataTypeScalingMode=Specify via dialog  OutDataTypeStr=fixdt('double')  DoSatur=off
  Product : Product
  Redution_factor : Constant  Value=[0.8 0.85 0.88 0.95 1 0.98 0.95]
  SOCEstimator : Subsystem  TreatAsAtomicUnit=on
  SOC_Mapping : Subsystem
  Scope : Scope
  Scope1 : Scope
  Scope2 : Scope
  Subsystem : Subsystem
  Temp : Constant  Value=[0 10 20 30 40 50 60]
  Cell_Voltage : Outport
  Cell_temp : Outport  Port=2
  wires:
  2RC/2(V2) -> Add/2
  SOC_Mapping/3(C1) -> 2RC/4(C1)
  SOCEstimator/1(SOC) -> SOC_Mapping/1(SOC), Scope/1
  Add/1 -> Scope2/1, Cell_Voltage/1
  SOC_Mapping/1(Ri) -> Subsystem/2(Ri), 2RC/2(Ri)
  2RC/1(V1) -> Add/1
  2RC/3(Vi) -> Add/3
  Cell_Current/1 -> Subsystem/1(Cell_Current), 2RC/1(Current), SOCEstimator/2(Current)
  SOC_Mapping/2(R1) -> 2RC/3(R1)
  [Cell_Capacity] -> Product/1
  SOC_Mapping/5(C2) -> 2RC/6(C2)
  SOC_Mapping/4(R2) -> 2RC/5(R2)
  [SOC_Iinitial] -> SOCEstimator/1(SOC_Initial)
  SOC_Mapping/6(OCV) -> Add/4
  Subsystem/1(Temp_Cell) -> Scope1/1, SOC_Mapping/2(Cell_Temp), Lookup Table Dynamic2/1, Cell_temp/1
  Product/1 -> SOCEstimator/3(Cell_Capacity)
  Lookup Table Dynamic2/1 -> Product/2
  Temp/1 -> Lookup Table Dynamic2/2
  Redution_factor/1 -> Lookup Table Dynamic2/3

== system Final_Dual1/Battery1/Module2/SubModule_5/Cell9 ==
  Cell_Current : Inport
  2RC : Subsystem
  Add : Sum  Inputs=---+
  Lookup Table Dynamic2 : simulink/Lookup Tables/Lookup Table Dynamic  LookUpMeth=Interpolation-Use End Values  OutDataType=fixdt('double')  OutScaling=[]  OutputDataTypeScalingMode=Specify via dialog  OutDataTypeStr=fixdt('double')  DoSatur=off
  Product : Product
  Redution_factor : Constant  Value=[0.8 0.85 0.88 0.95 1 0.98 0.95]
  SOCEstimator : Subsystem  TreatAsAtomicUnit=on
  SOC_Mapping : Subsystem
  Scope : Scope
  Scope1 : Scope
  Scope2 : Scope
  Subsystem : Subsystem
  Temp : Constant  Value=[0 10 20 30 40 50 60]
  Cell_Voltage : Outport
  Cell_temp : Outport  Port=2
  wires:
  Redution_factor/1 -> Lookup Table Dynamic2/3
  Temp/1 -> Lookup Table Dynamic2/2
  Lookup Table Dynamic2/1 -> Product/2
  Product/1 -> SOCEstimator/3(Cell_Capacity)
  Subsystem/1(Temp_Cell) -> Cell_temp/1, Lookup Table Dynamic2/1, SOC_Mapping/2(Cell_Temp), Scope1/1
  SOC_Mapping/6(OCV) -> Add/4
  [SOC_Iinitial] -> SOCEstimator/1(SOC_Initial)
  SOC_Mapping/4(R2) -> 2RC/5(R2)
  SOC_Mapping/5(C2) -> 2RC/6(C2)
  [Cell_Capacity] -> Product/1
  SOC_Mapping/2(R1) -> 2RC/3(R1)
  Cell_Current/1 -> SOCEstimator/2(Current), 2RC/1(Current), Subsystem/1(Cell_Current)
  2RC/3(Vi) -> Add/3
  2RC/1(V1) -> Add/1
  SOC_Mapping/1(Ri) -> 2RC/2(Ri), Subsystem/2(Ri)
  Add/1 -> Cell_Voltage/1, Scope2/1
  SOCEstimator/1(SOC) -> Scope/1, SOC_Mapping/1(SOC)
  SOC_Mapping/3(C1) -> 2RC/4(C1)
  2RC/2(V2) -> Add/2

== system Final_Dual1/Battery1/Module2/SubModule_6/Cell1 ==
  Cell_Current : Inport
  2RC : Subsystem
  Add : Sum  Inputs=---+
  Lookup Table Dynamic2 : simulink/Lookup Tables/Lookup Table Dynamic  LookUpMeth=Interpolation-Use End Values  OutDataType=fixdt('double')  OutScaling=[]  OutputDataTypeScalingMode=Specify via dialog  OutDataTypeStr=fixdt('double')  DoSatur=off
  Product : Product
  Redution_factor : Constant  Value=[0.8 0.85 0.88 0.95 1 0.98 0.95]
  SOCEstimator : Subsystem  TreatAsAtomicUnit=on
  SOC_Mapping : Subsystem
  Scope : Scope
  Scope1 : Scope
  Scope2 : Scope
  Subsystem : Subsystem
  Temp : Constant  Value=[0 10 20 30 40 50 60]
  Cell_Voltage : Outport
  Cell_temp : Outport  Port=2
  wires:
  Redution_factor/1 -> Lookup Table Dynamic2/3
  Temp/1 -> Lookup Table Dynamic2/2
  Lookup Table Dynamic2/1 -> Product/2
  Product/1 -> SOCEstimator/3(Cell_Capacity)
  Subsystem/1(Temp_Cell) -> Cell_temp/1, Lookup Table Dynamic2/1, SOC_Mapping/2(Cell_Temp), Scope1/1
  SOC_Mapping/6(OCV) -> Add/4
  [SOC_Iinitial] -> SOCEstimator/1(SOC_Initial)
  SOC_Mapping/4(R2) -> 2RC/5(R2)
  SOC_Mapping/5(C2) -> 2RC/6(C2)
  [Cell_Capacity] -> Product/1
  SOC_Mapping/2(R1) -> 2RC/3(R1)
  Cell_Current/1 -> SOCEstimator/2(Current), 2RC/1(Current), Subsystem/1(Cell_Current)
  2RC/3(Vi) -> Add/3
  2RC/1(V1) -> Add/1
  SOC_Mapping/1(Ri) -> 2RC/2(Ri), Subsystem/2(Ri)
  Add/1 -> Cell_Voltage/1, Scope2/1
  SOCEstimator/1(SOC) -> Scope/1, SOC_Mapping/1(SOC)
  SOC_Mapping/3(C1) -> 2RC/4(C1)
  2RC/2(V2) -> Add/2

== system Final_Dual1/Battery1/Module2/SubModule_6/Cell10 ==
  Cell_Current : Inport
  2RC : Subsystem
  Add : Sum  Inputs=---+
  Lookup Table Dynamic2 : simulink/Lookup Tables/Lookup Table Dynamic  LookUpMeth=Interpolation-Use End Values  OutDataType=fixdt('double')  OutScaling=[]  OutputDataTypeScalingMode=Specify via dialog  OutDataTypeStr=fixdt('double')  DoSatur=off
  Product : Product
  Redution_factor : Constant  Value=[0.8 0.85 0.88 0.95 1 0.98 0.95]
  SOCEstimator : Subsystem  TreatAsAtomicUnit=on
  SOC_Mapping : Subsystem
  Scope : Scope
  Scope1 : Scope
  Scope2 : Scope
  Subsystem : Subsystem
  Temp : Constant  Value=[0 10 20 30 40 50 60]
  Cell_Voltage : Outport
  Cell_temp : Outport  Port=2
  wires:
  Redution_factor/1 -> Lookup Table Dynamic2/3
  Temp/1 -> Lookup Table Dynamic2/2
  Lookup Table Dynamic2/1 -> Product/2
  Product/1 -> SOCEstimator/3(Cell_Capacity)
  Subsystem/1(Temp_Cell) -> Cell_temp/1, Lookup Table Dynamic2/1, SOC_Mapping/2(Cell_Temp), Scope1/1
  SOC_Mapping/6(OCV) -> Add/4
  [SOC_Iinitial] -> SOCEstimator/1(SOC_Initial)
  SOC_Mapping/4(R2) -> 2RC/5(R2)
  SOC_Mapping/5(C2) -> 2RC/6(C2)
  [Cell_Capacity] -> Product/1
  SOC_Mapping/2(R1) -> 2RC/3(R1)
  Cell_Current/1 -> SOCEstimator/2(Current), 2RC/1(Current), Subsystem/1(Cell_Current)
  2RC/3(Vi) -> Add/3
  2RC/1(V1) -> Add/1
  SOC_Mapping/1(Ri) -> 2RC/2(Ri), Subsystem/2(Ri)
  Add/1 -> Cell_Voltage/1, Scope2/1
  SOCEstimator/1(SOC) -> Scope/1, SOC_Mapping/1(SOC)
  SOC_Mapping/3(C1) -> 2RC/4(C1)
  2RC/2(V2) -> Add/2

== system Final_Dual1/Battery1/Module2/SubModule_6/Cell11 ==
  Cell_Current : Inport
  2RC : Subsystem
  Add : Sum  Inputs=---+
  Lookup Table Dynamic2 : simulink/Lookup Tables/Lookup Table Dynamic  LookUpMeth=Interpolation-Use End Values  OutDataType=fixdt('double')  OutScaling=[]  OutputDataTypeScalingMode=Specify via dialog  OutDataTypeStr=fixdt('double')  DoSatur=off
  Product : Product
  Redution_factor : Constant  Value=[0.8 0.85 0.88 0.95 1 0.98 0.95]
  SOCEstimator : Subsystem  TreatAsAtomicUnit=on
  SOC_Mapping : Subsystem
  Scope : Scope
  Scope1 : Scope
  Scope2 : Scope
  Subsystem : Subsystem
  Temp : Constant  Value=[0 10 20 30 40 50 60]
  Cell_Voltage : Outport
  Cell_temp : Outport  Port=2
  wires:
  2RC/2(V2) -> Add/2
  SOC_Mapping/3(C1) -> 2RC/4(C1)
  SOCEstimator/1(SOC) -> SOC_Mapping/1(SOC), Scope/1
  Add/1 -> Scope2/1, Cell_Voltage/1
  SOC_Mapping/1(Ri) -> Subsystem/2(Ri), 2RC/2(Ri)
  2RC/1(V1) -> Add/1
  2RC/3(Vi) -> Add/3
  Cell_Current/1 -> Subsystem/1(Cell_Current), 2RC/1(Current), SOCEstimator/2(Current)
  SOC_Mapping/2(R1) -> 2RC/3(R1)
  [Cell_Capacity] -> Product/1
  SOC_Mapping/5(C2) -> 2RC/6(C2)
  SOC_Mapping/4(R2) -> 2RC/5(R2)
  [SOC_Iinitial] -> SOCEstimator/1(SOC_Initial)
  SOC_Mapping/6(OCV) -> Add/4
  Subsystem/1(Temp_Cell) -> Scope1/1, SOC_Mapping/2(Cell_Temp), Lookup Table Dynamic2/1, Cell_temp/1
  Product/1 -> SOCEstimator/3(Cell_Capacity)
  Lookup Table Dynamic2/1 -> Product/2
  Temp/1 -> Lookup Table Dynamic2/2
  Redution_factor/1 -> Lookup Table Dynamic2/3

== system Final_Dual1/Battery1/Module2/SubModule_6/Cell12 ==
  Cell_Current : Inport
  2RC : Subsystem
  Add : Sum  Inputs=---+
  Lookup Table Dynamic2 : simulink/Lookup Tables/Lookup Table Dynamic  LookUpMeth=Interpolation-Use End Values  OutDataType=fixdt('double')  OutScaling=[]  OutputDataTypeScalingMode=Specify via dialog  OutDataTypeStr=fixdt('double')  DoSatur=off
  Product : Product
  Redution_factor : Constant  Value=[0.8 0.85 0.88 0.95 1 0.98 0.95]
  SOCEstimator : Subsystem  TreatAsAtomicUnit=on
  SOC_Mapping : Subsystem
  Scope : Scope
  Scope1 : Scope
  Scope2 : Scope
  Subsystem : Subsystem
  Temp : Constant  Value=[0 10 20 30 40 50 60]
  Cell_Voltage : Outport
  Cell_temp : Outport  Port=2
  wires:
  Redution_factor/1 -> Lookup Table Dynamic2/3
  Temp/1 -> Lookup Table Dynamic2/2
  Lookup Table Dynamic2/1 -> Product/2
  Product/1 -> SOCEstimator/3(Cell_Capacity)
  Subsystem/1(Temp_Cell) -> Cell_temp/1, Lookup Table Dynamic2/1, SOC_Mapping/2(Cell_Temp), Scope1/1
  SOC_Mapping/6(OCV) -> Add/4
  [SOC_Iinitial] -> SOCEstimator/1(SOC_Initial)
  SOC_Mapping/4(R2) -> 2RC/5(R2)
  SOC_Mapping/5(C2) -> 2RC/6(C2)
  [Cell_Capacity] -> Product/1
  SOC_Mapping/2(R1) -> 2RC/3(R1)
  Cell_Current/1 -> SOCEstimator/2(Current), 2RC/1(Current), Subsystem/1(Cell_Current)
  2RC/3(Vi) -> Add/3
  2RC/1(V1) -> Add/1
  SOC_Mapping/1(Ri) -> 2RC/2(Ri), Subsystem/2(Ri)
  Add/1 -> Cell_Voltage/1, Scope2/1
  SOCEstimator/1(SOC) -> Scope/1, SOC_Mapping/1(SOC)
  SOC_Mapping/3(C1) -> 2RC/4(C1)
  2RC/2(V2) -> Add/2

== system Final_Dual1/Battery1/Module2/SubModule_6/Cell13 ==
  Cell_Current : Inport
  2RC : Subsystem
  Add : Sum  Inputs=---+
  Lookup Table Dynamic2 : simulink/Lookup Tables/Lookup Table Dynamic  LookUpMeth=Interpolation-Use End Values  OutDataType=fixdt('double')  OutScaling=[]  OutputDataTypeScalingMode=Specify via dialog  OutDataTypeStr=fixdt('double')  DoSatur=off
  Product : Product
  Redution_factor : Constant  Value=[0.8 0.85 0.88 0.95 1 0.98 0.95]
  SOCEstimator : Subsystem  TreatAsAtomicUnit=on
  SOC_Mapping : Subsystem
  Scope : Scope
  Scope1 : Scope
  Scope2 : Scope
  Subsystem : Subsystem
  Temp : Constant  Value=[0 10 20 30 40 50 60]
  Cell_Voltage : Outport
  Cell_temp : Outport  Port=2
  wires:
  2RC/2(V2) -> Add/2
  SOC_Mapping/3(C1) -> 2RC/4(C1)
  SOCEstimator/1(SOC) -> SOC_Mapping/1(SOC), Scope/1
  Add/1 -> Scope2/1, Cell_Voltage/1
  SOC_Mapping/1(Ri) -> Subsystem/2(Ri), 2RC/2(Ri)
  2RC/1(V1) -> Add/1
  2RC/3(Vi) -> Add/3
  Cell_Current/1 -> Subsystem/1(Cell_Current), 2RC/1(Current), SOCEstimator/2(Current)
  SOC_Mapping/2(R1) -> 2RC/3(R1)
  [Cell_Capacity] -> Product/1
  SOC_Mapping/5(C2) -> 2RC/6(C2)
  SOC_Mapping/4(R2) -> 2RC/5(R2)
  [SOC_Iinitial] -> SOCEstimator/1(SOC_Initial)
  SOC_Mapping/6(OCV) -> Add/4
  Subsystem/1(Temp_Cell) -> Scope1/1, SOC_Mapping/2(Cell_Temp), Lookup Table Dynamic2/1, Cell_temp/1
  Product/1 -> SOCEstimator/3(Cell_Capacity)
  Lookup Table Dynamic2/1 -> Product/2
  Temp/1 -> Lookup Table Dynamic2/2
  Redution_factor/1 -> Lookup Table Dynamic2/3

== system Final_Dual1/Battery1/Module2/SubModule_6/Cell14 ==
  Cell_Current : Inport
  2RC : Subsystem
  Add : Sum  Inputs=---+
  Lookup Table Dynamic2 : simulink/Lookup Tables/Lookup Table Dynamic  LookUpMeth=Interpolation-Use End Values  OutDataType=fixdt('double')  OutScaling=[]  OutputDataTypeScalingMode=Specify via dialog  OutDataTypeStr=fixdt('double')  DoSatur=off
  Product : Product
  Redution_factor : Constant  Value=[0.8 0.85 0.88 0.95 1 0.98 0.95]
  SOCEstimator : Subsystem  TreatAsAtomicUnit=on
  SOC_Mapping : Subsystem
  Scope : Scope
  Scope1 : Scope
  Scope2 : Scope
  Subsystem : Subsystem
  Temp : Constant  Value=[0 10 20 30 40 50 60]
  Cell_Voltage : Outport
  Cell_temp : Outport  Port=2
  wires:
  2RC/2(V2) -> Add/2
  SOC_Mapping/3(C1) -> 2RC/4(C1)
  SOCEstimator/1(SOC) -> SOC_Mapping/1(SOC), Scope/1
  Add/1 -> Scope2/1, Cell_Voltage/1
  SOC_Mapping/1(Ri) -> Subsystem/2(Ri), 2RC/2(Ri)
  2RC/1(V1) -> Add/1
  2RC/3(Vi) -> Add/3
  Cell_Current/1 -> Subsystem/1(Cell_Current), 2RC/1(Current), SOCEstimator/2(Current)
  SOC_Mapping/2(R1) -> 2RC/3(R1)
  [Cell_Capacity] -> Product/1
  SOC_Mapping/5(C2) -> 2RC/6(C2)
  SOC_Mapping/4(R2) -> 2RC/5(R2)
  [SOC_Iinitial] -> SOCEstimator/1(SOC_Initial)
  SOC_Mapping/6(OCV) -> Add/4
  Subsystem/1(Temp_Cell) -> Scope1/1, SOC_Mapping/2(Cell_Temp), Lookup Table Dynamic2/1, Cell_temp/1
  Product/1 -> SOCEstimator/3(Cell_Capacity)
  Lookup Table Dynamic2/1 -> Product/2
  Temp/1 -> Lookup Table Dynamic2/2
  Redution_factor/1 -> Lookup Table Dynamic2/3

== system Final_Dual1/Battery1/Module2/SubModule_6/Cell15 ==
  Cell_Current : Inport
  2RC : Subsystem
  Add : Sum  Inputs=---+
  Lookup Table Dynamic2 : simulink/Lookup Tables/Lookup Table Dynamic  LookUpMeth=Interpolation-Use End Values  OutDataType=fixdt('double')  OutScaling=[]  OutputDataTypeScalingMode=Specify via dialog  OutDataTypeStr=fixdt('double')  DoSatur=off
  Product : Product
  Redution_factor : Constant  Value=[0.8 0.85 0.88 0.95 1 0.98 0.95]
  SOCEstimator : Subsystem  TreatAsAtomicUnit=on
  SOC_Mapping : Subsystem
  Scope : Scope
  Scope1 : Scope
  Scope2 : Scope
  Subsystem : Subsystem
  Temp : Constant  Value=[0 10 20 30 40 50 60]
  Cell_Voltage : Outport
  Cell_temp : Outport  Port=2
  wires:
  2RC/2(V2) -> Add/2
  SOC_Mapping/3(C1) -> 2RC/4(C1)
  SOCEstimator/1(SOC) -> SOC_Mapping/1(SOC), Scope/1
  Add/1 -> Scope2/1, Cell_Voltage/1
  SOC_Mapping/1(Ri) -> Subsystem/2(Ri), 2RC/2(Ri)
  2RC/1(V1) -> Add/1
  2RC/3(Vi) -> Add/3
  Cell_Current/1 -> Subsystem/1(Cell_Current), 2RC/1(Current), SOCEstimator/2(Current)
  SOC_Mapping/2(R1) -> 2RC/3(R1)
  [Cell_Capacity] -> Product/1
  SOC_Mapping/5(C2) -> 2RC/6(C2)
  SOC_Mapping/4(R2) -> 2RC/5(R2)
  [SOC_Iinitial] -> SOCEstimator/1(SOC_Initial)
  SOC_Mapping/6(OCV) -> Add/4
  Subsystem/1(Temp_Cell) -> Scope1/1, SOC_Mapping/2(Cell_Temp), Lookup Table Dynamic2/1, Cell_temp/1
  Product/1 -> SOCEstimator/3(Cell_Capacity)
  Lookup Table Dynamic2/1 -> Product/2
  Temp/1 -> Lookup Table Dynamic2/2
  Redution_factor/1 -> Lookup Table Dynamic2/3

== system Final_Dual1/Battery1/Module2/SubModule_6/Cell16 ==
  Cell_Current : Inport
  2RC : Subsystem
  Add : Sum  Inputs=---+
  Lookup Table Dynamic2 : simulink/Lookup Tables/Lookup Table Dynamic  LookUpMeth=Interpolation-Use End Values  OutDataType=fixdt('double')  OutScaling=[]  OutputDataTypeScalingMode=Specify via dialog  OutDataTypeStr=fixdt('double')  DoSatur=off
  Product : Product
  Redution_factor : Constant  Value=[0.8 0.85 0.88 0.95 1 0.98 0.95]
  SOCEstimator : Subsystem  TreatAsAtomicUnit=on
  SOC_Mapping : Subsystem
  Scope : Scope
  Scope1 : Scope
  Scope2 : Scope
  Subsystem : Subsystem
  Temp : Constant  Value=[0 10 20 30 40 50 60]
  Cell_Voltage : Outport
  Cell_temp : Outport  Port=2
  wires:
  2RC/2(V2) -> Add/2
  SOC_Mapping/3(C1) -> 2RC/4(C1)
  SOCEstimator/1(SOC) -> SOC_Mapping/1(SOC), Scope/1
  Add/1 -> Scope2/1, Cell_Voltage/1
  SOC_Mapping/1(Ri) -> Subsystem/2(Ri), 2RC/2(Ri)
  2RC/1(V1) -> Add/1
  2RC/3(Vi) -> Add/3
  Cell_Current/1 -> Subsystem/1(Cell_Current), 2RC/1(Current), SOCEstimator/2(Current)
  SOC_Mapping/2(R1) -> 2RC/3(R1)
  [Cell_Capacity] -> Product/1
  SOC_Mapping/5(C2) -> 2RC/6(C2)
  SOC_Mapping/4(R2) -> 2RC/5(R2)
  [SOC_Iinitial] -> SOCEstimator/1(SOC_Initial)
  SOC_Mapping/6(OCV) -> Add/4
  Subsystem/1(Temp_Cell) -> Scope1/1, SOC_Mapping/2(Cell_Temp), Lookup Table Dynamic2/1, Cell_temp/1
  Product/1 -> SOCEstimator/3(Cell_Capacity)
  Lookup Table Dynamic2/1 -> Product/2
  Temp/1 -> Lookup Table Dynamic2/2
  Redution_factor/1 -> Lookup Table Dynamic2/3

== system Final_Dual1/Battery1/Module2/SubModule_6/Cell17 ==
  Cell_Current : Inport
  2RC : Subsystem
  Add : Sum  Inputs=---+
  Lookup Table Dynamic2 : simulink/Lookup Tables/Lookup Table Dynamic  LookUpMeth=Interpolation-Use End Values  OutDataType=fixdt('double')  OutScaling=[]  OutputDataTypeScalingMode=Specify via dialog  OutDataTypeStr=fixdt('double')  DoSatur=off
  Product : Product
  Redution_factor : Constant  Value=[0.8 0.85 0.88 0.95 1 0.98 0.95]
  SOCEstimator : Subsystem  TreatAsAtomicUnit=on
  SOC_Mapping : Subsystem
  Scope : Scope
  Scope1 : Scope
  Scope2 : Scope
  Subsystem : Subsystem
  Temp : Constant  Value=[0 10 20 30 40 50 60]
  Cell_Voltage : Outport
  Cell_temp : Outport  Port=2
  wires:
  Redution_factor/1 -> Lookup Table Dynamic2/3
  Temp/1 -> Lookup Table Dynamic2/2
  Lookup Table Dynamic2/1 -> Product/2
  Product/1 -> SOCEstimator/3(Cell_Capacity)
  Subsystem/1(Temp_Cell) -> Cell_temp/1, Lookup Table Dynamic2/1, SOC_Mapping/2(Cell_Temp), Scope1/1
  SOC_Mapping/6(OCV) -> Add/4
  [SOC_Iinitial] -> SOCEstimator/1(SOC_Initial)
  SOC_Mapping/4(R2) -> 2RC/5(R2)
  SOC_Mapping/5(C2) -> 2RC/6(C2)
  [Cell_Capacity] -> Product/1
  SOC_Mapping/2(R1) -> 2RC/3(R1)
  Cell_Current/1 -> SOCEstimator/2(Current), 2RC/1(Current), Subsystem/1(Cell_Current)
  2RC/3(Vi) -> Add/3
  2RC/1(V1) -> Add/1
  SOC_Mapping/1(Ri) -> 2RC/2(Ri), Subsystem/2(Ri)
  Add/1 -> Cell_Voltage/1, Scope2/1
  SOCEstimator/1(SOC) -> Scope/1, SOC_Mapping/1(SOC)
  SOC_Mapping/3(C1) -> 2RC/4(C1)
  2RC/2(V2) -> Add/2
